simulink model "simscape_101_simpleActuator"  (R2019a)
settings: Solver=VariableStepAuto  StartTime=0.0  StopTime=10.0  RelTol=1e-3  AbsTol=1e-3  EnableMultiTasking=on
libraries: fl_lib x7, nesl_utility x4, sh_lib x3, sdl_lib x1
settings Model: Creator=ashimahara  LastModifiedBy=ashimahara
settings SolverCC: AutoScaleAbsTol=off
settings DataIOCC: LimitDataPoints=on  MaxDataPoints=10000
settings OptimizationCC: LifeSpan=inf
settings DebuggingCC: AllowSymbolicDim=off  PregeneratedLibrarySubsystemCodeDiagnostic=none  SFUnexpectedBacktrackingDiag=warning  SFNoUnconditionalDefaultTransitionDiag=warning  SFExecutionAtInitializationDiag=none  ArithmeticOperatorsInVariantConditions=warning
settings SFSimCC: SimUseLocalCustomCode=off
settings RTWCC: RTWUseLocalCustomCode=off
settings CodeAppCC: StateflowObjectComments=on
settings GRTTargetCC: TargetLangStandard=C89/C90 (ANSI)  GeneratePreprocessorConditionals=Disable all
settings ConfigComp: CovMetricSettings=dw  CovHtmlReporting=on  CovSaveCumulativeToWorkspaceVar=on  CovSaveSingleToWorkspaceVar=on  CovExternalEMLEnable=off  CovSFcnEnable=off
settings SimscapeCC: SimscapeLogType=all  SimscapeLogDataHistory=10000

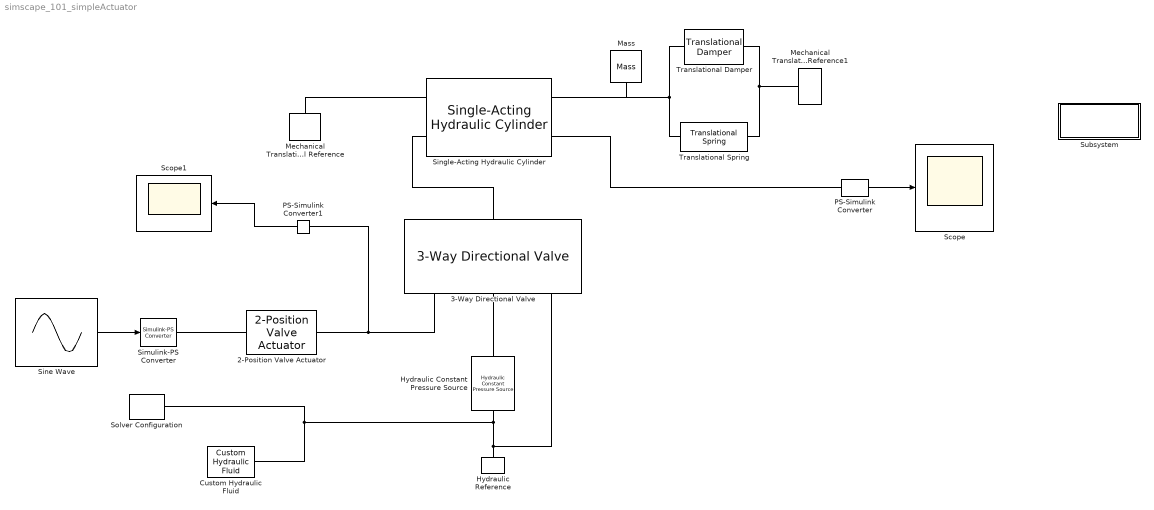
== system simscape_101_simpleActuator ==
  2-Position Valve Actuator : sh_lib/Valves/Valve Actuators/2-Position Valve Actuator  stroke=0.01 m  t_on=0.1 s  t_off=0.1 s  act_signal=24  init_position=0  act_orientation=1
      settings: SourceProductName=Simscape Fluids  SourceProductBaseCode=SH
  3-Way Directional Valve : sh_lib/Valves/Directional Valves/3-Way Directional Valve  area_spec=sh.valves.directional_valves.enum.area_spec.identical  x_0_P=0 m  x_0_T=0.01 m  mdl_type_identical=sh.valves.directional_valves.enum.mdl_type.linear  mdl_type_different=sh.valves.directional_valves.enum.mdl_type.linear  opening_max=0.005 m  area_max=0.5e-4 m^2  opening_max_P_A=0.005 m  area_max_P_A=0.5e-4 m^2  opening_max_A_T=0.005 m  area_max_A_T=0.5e-4 m^2  opening_area_tab=[-.002, 0, .002, .005, .015] m  area_tab=[1e-09, 2.0352e-07, 4.0736e-05, .00011438, .00034356] m^2  opening_flow_rate_tab=[-.002, 0, .002, .005, .015] m  pressure_tab=[-10000000, -5000000, -2000000, 2000000, 5000000, 10000000] Pa  flow_rate_tab=[-1e-07, -7.0711e-08, -4.4721e-08, 4.4721e-08, 7.0711e-08, 1e-07; -2.0352e-05, -1.4391e-05, -9.1017e-06, 9.1017e-06, 1.4391e-05, 2.0352e-05; -.0040736, -.0028805, -.0018218, .0018218, .0028805, .0040736; -.011438, -.0080879, -.0051152, .0051152, .0080879, .011438; -.034356, -.024293, -.015364, .015364, .024293, .034356] m^3/s  opening_area_tab_P_A=[-.002, 0, .002, .005, .015] m  area_tab_P_A=[1e-09, 2.0352e-07, 4.0736e-05, .00011438, .00034356] m^2  opening_flow_rate_tab_P_A=[-.002, 0, .002, .005, .015] m  pressure_tab_P_A=[-10000000, -5000000, -2000000, 2000000, 5000000, 10000000] Pa  flow_rate_tab_P_A=[-1e-07, -7.0711e-08, -4.4721e-08, 4.4721e-08, 7.0711e-08, 1e-07; -2.0352e-05, -1.4391e-05, -9.1017e-06, 9.1017e-06, 1.4391e-05, 2.0352e-05; -.0040736, -.0028805, -.0018218, .0018218, .0028805, .0040736; -.011438, -.0080879, -.0051152, .0051152, .0080879, .011438; -.034356, -.024293, -.015364, .015364, .024293, .034356] m^3/s  opening_area_tab_A_T=[-.002, 0, .002, .005, .015] m  area_tab_A_T=[1e-09, 2.0352e-07, 4.0736e-05, .00011438, .00034356] m^2  opening_flow_rate_tab_A_T=[-.002, 0, .002, .005, .015] m  pressure_tab_A_T=[-10000000, -5000000, -2000000, 2000000, 5000000, 10000000] Pa  flow_rate_tab_A_T=[-1e-07, -7.0711e-08, -4.4721e-08, 4.4721e-08, 7.0711e-08, 1e-07; -2.0352e-05, -1.4391e-05, -9.1017e-06, 9.1017e-06, 1.4391e-05, 2.0352e-05; -.0040736, -.0028805, -.0018218, .0018218, .0028805, .0040736; -.011438, -.0080879, -.0051152, .0051152, .0080879, .011438; -.034356, -.024293, -.015364, .015364, .024293, .034356] m^3/s  interp_method_identical=sh.valves.directional_valves.enum.interp_method.linear  interp_method_different=sh.valves.directional_valves.enum.interp_method.linear  extrap_method_identical=sh.valves.directional_valves.enum.extrap_method.linear  extrap_method_different=sh.valves.directional_valves.enum.extrap_method.linear  A_leak=1e-12 m^2  C_d=0.7  lam_spec=sh.valves.directional_valves.enum.lam_spec.pressure_ratio  B_lam=0.999  Re_cr=12
      settings: SourceProductName=Simscape Fluids  SourceProductBaseCode=SH
  Custom Hydraulic Fluid : fl_lib/Hydraulic/Hydraulic Utilities/Custom Hydraulic Fluid  density=850 kg/m^3  viscosity_kin=18e-6 m^2/s  bulk=0.8e9 Pa  alpha=0.005  range_error=2
      settings: SourceProductName=Simscape  SourceProductBaseCode=SS
  Hydraulic Constant Pressure Source : fl_lib/Hydraulic/Hydraulic Sources/Hydraulic Constant Pressure Source  commanded_pressure=10e5 Pa
      settings: SourceProductName=Simscape  SourceProductBaseCode=SS
  Hydraulic Reference : fl_lib/Hydraulic/Hydraulic Elements/Hydraulic Reference
      settings: SourceProductName=Simscape
  Mass : fl_lib/Mechanical/Translational Elements/Mass  mass=1 kg  v_specify=off  v_priority=High  v=0 m/s  v_nominal_specify=off  v_nominal_unit=m/s  v_nominal_value=1  f_specify=off  f_priority=None  f=0 N  f_nominal_specify=off  f_nominal_unit=N  f_nominal_value=1
  Mechanical Translational Reference : fl_lib/Mechanical/Translational Elements/Mechanical Translational Reference
  Mechanical Translational Reference1 : fl_lib/Mechanical/Translational Elements/Mechanical Translational Reference
  PS-Simulink Converter : nesl_utility/PS-Simulink Converter  PhysicalDomain=network_engine_domain  SubClassName=ps_output  LeftPortType=input  RightPortType=output  PseudoPeriodic=off  Frequencies=[]  Unit=1  AffineConversion=off
  PS-Simulink Converter1 : nesl_utility/PS-Simulink Converter  PhysicalDomain=network_engine_domain  SubClassName=ps_output  LeftPortType=input  RightPortType=output  PseudoPeriodic=off  Frequencies=[]  Unit=1  AffineConversion=off
  Scope : Scope
  Scope1 : Scope
  Simulink-PS Converter : nesl_utility/Simulink-PS Converter  PhysicalDomain=network_engine_domain  SubClassName=ps_input  LeftPortType=input  RightPortType=output  PseudoPeriodic=off  Frequencies=[]  NoiseDistribution=none  NoiseParameters=[]  Unit=1  AffineConversion=off  FilteringAndDerivatives=provide  SimscapeFilterOrder=1  InputFilterTimeConstant=0.001  UdotUserProvided=0
  Sine Wave : Sin  Amplitude=24  SampleTime=0
  Single-Acting Hydraulic Cylinder : sh_lib/Hydraulic Cylinders/Single-Acting Hydraulic Cylinder  area=1e-3 m^2  stroke=0.1 m  init_pos=0 m  dead_vol=1e-4 m^3  init_pressure=0 Pa  k_sh=1.4  stiff=1e6 N/m  D=150 N/(m/s)  hardstop_model=1  transition=0.1 mm  or=1
      settings: SourceProductName=Simscape Fluids  SourceProductBaseCode=SH
  Solver Configuration : nesl_utility/Solver Configuration  PhysicalDomain=network_engine_domain  SubClassName=solver  LeftPortType=input  RightPortType=generic  Tones=[]  Harmonics=[]  SimulateNoise=off  Profile=off  UseLocalSampling=off  EnableSwitchedLinearOptims=on  FrequencyDomain=off  UseCCode=off  RelTol=0.001  AbsTol=1e-06  MinStep=1e-09  ToWorkspace=off  RevertToSquareIcSolve=off  NumHomotopyIterations=100  PhasorMode=off  PhasorModeNumHarmonics=1  DoDC=off  ResidualTolerance=1e-09  UseLocalSolver=off  LocalSolverChoice=NE_BACKWARD_EULER_ADVANCER  LocalSolverSampleTime=0.001  DoFixedCost=off  MaxNonlinIter=3  MaxModeIter=2  LinearAlgebra=auto  EquationFormulation=NE_TIME_EF  DelaysMemoryBudget=1024  AutomaticFiltering=on  FilteringTimeConstant=0.001  PartitionStorageMethod=AS_NEEDED  PartitionMemoryBudget=1024  PartitionMethod=ROBUST
  Subsystem : Subsystem
      settings: OpenFcn=open_system('simscape')
      mask Display: disp(sprintf('Open Simscape\nLibrary'));
  Translational Damper : sdl_lib/Couplings & Drives/Springs & Dampers/Translational Damper  D=10 N/(m/s)  enable_faults=0  b_fault=1e6 N/(m/s)  temporal_fault=0  fault_time=5 s  shock_fault=0  acceleration_limit=100 m/s^2  shock_limit=1  report_fault=1
      settings: SourceProductName=Simscape Driveline  SourceProductBaseCode=LD
  Translational Spring : fl_lib/Mechanical/Translational Elements/Translational Spring  spr_rate=250 N/m  v_specify=off  v_priority=None  v=0 m/s  v_nominal_specify=off  v_nominal_unit=m/s  v_nominal_value=1  f_specify=off  f_priority=None  f=0 N  f_nominal_specify=off  f_nominal_unit=N  f_nominal_value=1  x_specify=off  x_priority=High  x=0 m  x_nominal_specify=off  x_nominal_unit=m  x_nominal_value=1
  wires:
  PS-Simulink Converter/1 -> Scope/1
  Sine Wave/1 -> Simulink-PS Converter/1
  PS-Simulink Converter1/1 -> Scope1/1
  connections:
  Hydraulic Constant Pressure Source/RConn1 -- Solver Configuration/RConn1 -- Custom Hydraulic Fluid/RConn1 -- 3-Way Directional Valve/RConn3 -- Hydraulic Reference/LConn1
  Hydraulic Constant Pressure Source/LConn1 -- 3-Way Directional Valve/RConn2
  2-Position Valve Actuator/RConn1 -- PS-Simulink Converter1/LConn1 -- 3-Way Directional Valve/RConn1
  3-Way Directional Valve/LConn1 -- Single-Acting Hydraulic Cylinder/LConn2
  Mechanical Translational Reference/LConn1 -- Single-Acting Hydraulic Cylinder/LConn1
  Translational Damper/RConn1 -- Mechanical Translational Reference1/LConn1 -- Translational Spring/RConn1
  Translational Damper/LConn1 -- Mass/LConn1 -- Single-Acting Hydraulic Cylinder/RConn1 -- Translational Spring/LConn1
  Simulink-PS Converter/RConn1 -- 2-Position Valve Actuator/LConn1
  Single-Acting Hydraulic Cylinder/RConn2 -- PS-Simulink Converter/LConn1

== system simscape_101_simpleActuator/Subsystem ==
